simulink model "test_on_intes_cross2018_TestCase"  (R2018b)
settings: Solver=ode1  StartTime=0.0  StopTime=0  FixedStep=0.01  RelTol=1e-3
PostLoadFcn:
  | , if any(exist('dsrtsu_mdlpostloadfcn', 'file') == [2, 3, 6]), try dsrtsu_mdlpostloadfcn('Execute', bdroot); catch fprintf('Error in PostLoadFcn (dsrtsu_mdlpostloadfcn) for model "%s":\n %s\n', bdroot, lasterr); end, end,
values from neighbouring files (symbols this model uses):
  dt = 0.01    [test_on_intes_cross_Autotest.m]    (also in test_on_intes_cross_Autotest_Full.m)
undefined symbols (not defined in the file or in its folder): d0, v0
Description:
  | Standard RTI1401 template.
  | Supported MATLAB version:  R2018b.
settings Model: Tag=RTI1401  DSRTSU_INTERNAL_RTI_VER=540  DSRTSU_INTERNAL_RTI_TYPE=rti1401  RTICANMMDATA=struct('GeneralSetupData',struct('modelroot','C:\Users\linqi\Desktop\matlab\ACC\CarMaker\src_cm4sl','generalsettings',struct('filesettings',struct('destfolder',struct('Name','RTICANMM_FILES','Check',1),'buildfolder',struct('Name','.','Check',1),'AbsDestfolder',struct('Name','C:\Users\linqi\Desktop\matlab\ACC\CarMaker\src_cm4sl\RTICANMM_FILES'),'AbsBuildfolder',struct('Name','C:\Users\linqi\Desktop\matlab\ACC\CarMaker\src_cm4sl'))),'options',struct('addpaths',1,'rmpaths',1,'addtrcexclusion',logical(1),'cannavigator',struct('checkmonitoring',0),'show_usrtrc',0,'use_usrtrc',0),'advanced',struct('options',ones(1,100)),'MPSetup',{{}},'RTI',struct('Type','RTI1401','Ver','7.12','Date','02-May-2019'),'modelname','','block','untitled'))  DSRTSU_INTERNAL_RTIFPGA=130  Creator=linqi  LastModifiedBy=linqi
settings OptimizationCC: BlockReduction=off  OptimizeBlockIOStorage=off  BufferReuse=off  GlobalBufferReuse=off  ExpressionFolding=off  LocalBlockOutputs=off  OptimizeDataStoreBuffers=off  BusAssignmentInplaceUpdate=off
settings DebuggingCC: LibraryContextMissingDiagnostic=none
settings HardwareCC: ProdBitPerPointer=32  ProdBitPerSizeT=32  ProdBitPerPtrDiffT=32  ProdLargestAtomicInteger=Integer  ProdEndianess=BigEndian  ProdWordSize=32  ProdHWDeviceType=Custom Processor->Custom  TargetIntDivRoundTo=Zero  TargetEndianess=BigEndian  TargetHWDeviceType=Custom Processor->Custom
settings SFSimCC: SimUseLocalCustomCode=off  MATLABDynamicMemAlloc=off
settings RTWCC: SystemTargetFile=rti1401.tlc  MakeCommand=make_rti  TemplateMakefile=rti1401.tmf  Description=dSPACE DS1401 Hardware Platform  RTWUseLocalCustomCode=off
settings CodeAppCC: StateflowObjectComments=on
settings STFCustomTargetCC: ParMdlRefBuildCompliant=on  MatFileLogging=on  SystemTargetFile=rti1401.tlc
settings GRTTargetCC: TargetLangStandard=C89/C90 (ANSI)  CompOptLevelCompliant=off  ConcurrentExecutionCompliant=off  CombineOutputUpdateFcns=off  CPPClassGenCompliant=off  UseToolchainInfoCompliant=off
settings ConfigComp: CovMetricSettings=dswe

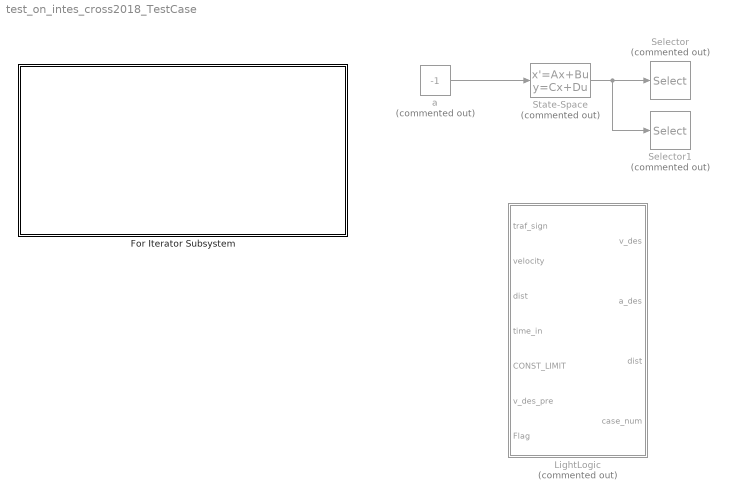
== system test_on_intes_cross2018_TestCase ==
  For Iterator Subsystem : Subsystem  TreatAsAtomicUnit=on
  LightLogic : MATLAB Function  Commented=on  TreatAsAtomicUnit=on
  Selector : Selector  Commented=on  IndexMode=Zero-based  InputPortWidth=2  IndexOptions=Index vector (dialog)  Indices=0  OutputSizes=1
  Selector1 : Selector  Commented=on  IndexMode=Zero-based  InputPortWidth=2  IndexOptions=Index vector (dialog)  Indices=1  OutputSizes=1
  State-Space : StateSpace  Commented=on  A=[0 1;0 0]  B=[0.01/2;1]  C=[1 0;0 1]  D=[0;0]  InitialCondition=[d0;v0]
  a : Constant  Commented=on  Value=-1
  wires:
  a/1 -> State-Space/1
  State-Space/1 -> Selector1/1, Selector/1

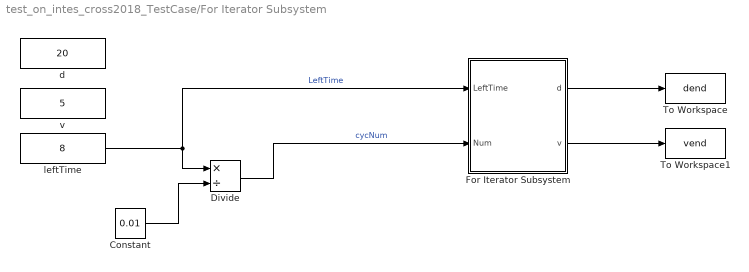
== system test_on_intes_cross2018_TestCase/For Iterator Subsystem ==
  Constant : Constant  Value=0.01  OutDataTypeStr=double
  Divide : Product  Inputs=*/
  For Iterator Subsystem : Subsystem  TreatAsAtomicUnit=on
  To Workspace : ToWorkspace  VariableName=dend  SaveFormat=Timeseries  SampleTime=-1
  To Workspace1 : ToWorkspace  VariableName=vend  SaveFormat=Timeseries  SampleTime=-1
  d : Constant  Value=20  OutDataTypeStr=double
  leftTime : Constant  Value=8  OutDataTypeStr=double
  v : Constant  Value=5  OutDataTypeStr=double
  wires:
  leftTime/1 -> For Iterator Subsystem/1(LeftTime), Divide/1  "LeftTime"
  Constant/1 -> Divide/2
  Divide/1 -> For Iterator Subsystem/2(Num)  "cycNum"
  For Iterator Subsystem/1(d) -> To Workspace/1
  For Iterator Subsystem/2(v) -> To Workspace1/1

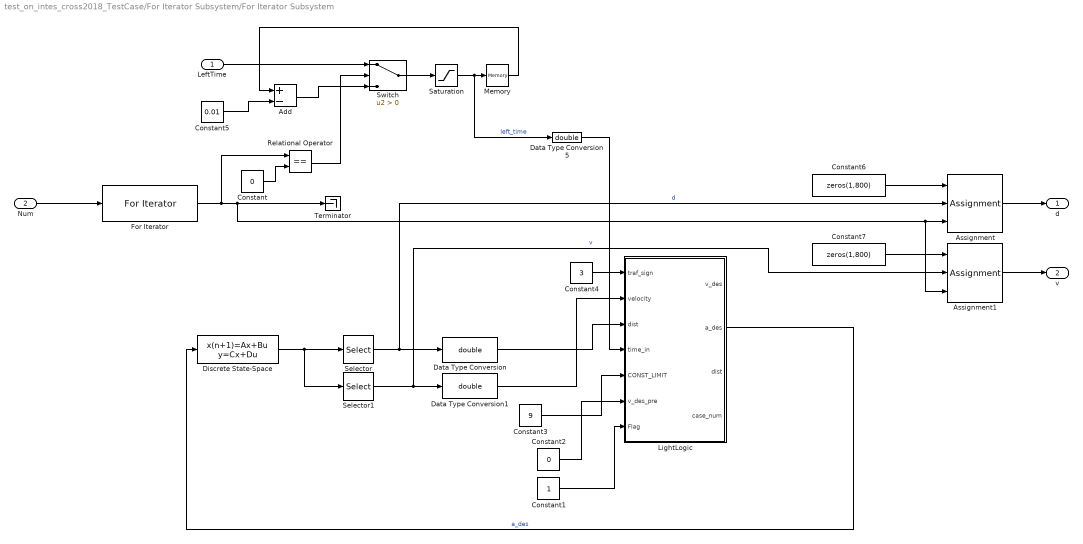
== system test_on_intes_cross2018_TestCase/For Iterator Subsystem/For Iterator Subsystem ==
  LeftTime : Inport
  Num : Inport  Port=2
  Add : Sum  Inputs=+-
  Assignment : Assignment  IndexMode=Zero-based  DiagnosticForDimensions=Warning  IndexOptions=Index vector (port)  Indices=1  OutputSizes=1
  Assignment1 : Assignment  IndexMode=Zero-based  DiagnosticForDimensions=Warning  IndexOptions=Index vector (port)  Indices=1  OutputSizes=1
  Constant : Constant  Value=0
  Constant1 : Constant  OutDataTypeStr=double
  Constant2 : Constant  Value=0  OutDataTypeStr=double
  Constant3 : Constant  Value=9  OutDataTypeStr=double
  Constant4 : Constant  Value=3  OutDataTypeStr=double
  Constant5 : Constant  Value=0.01
  Constant6 : Constant  Value=zeros(1,800)
  Constant7 : Constant  Value=zeros(1,800)
  Data Type Conversion : DataTypeConversion  OutDataTypeStr=double
  Data Type Conversion1 : DataTypeConversion  OutDataTypeStr=double
  Data Type Conversion5 : DataTypeConversion  OutDataTypeStr=double
  Discrete State-Space : DiscreteStateSpace  A=[1 -dt;0 1]  B=[-0.5*dt^2;dt]  C=[1 0;0 1]  D=[0;0]  InitialCondition=[d0;v0]  SampleTime=-1
  For Iterator : ForIterator  IterationSource=external  IndexMode=Zero-based
  LightLogic : MATLAB Function  TreatAsAtomicUnit=on
  Memory : Memory  InheritSampleTime=on
  Relational Operator : RelationalOperator  Operator===  OutDataTypeStr=boolean  RndMeth=Simplest
  Saturation : Saturate  UpperLimit=40  LowerLimit=0
  Selector : Selector  IndexMode=Zero-based  InputPortWidth=2  IndexOptions=Index vector (dialog)  Indices=0  OutputSizes=1
  Selector1 : Selector  IndexMode=Zero-based  InputPortWidth=2  IndexOptions=Index vector (dialog)  Indices=1  OutputSizes=1
  Switch : Switch  Criteria=u2 > Threshold
  Terminator : Terminator
  d : Outport
  v : Outport  Port=2
  wires:
  LightLogic/2(a_des) -> Discrete State-Space/1  "a_des"
  Discrete State-Space/1 -> Selector1/1, Selector/1
  Selector/1 -> Assignment/2, Data Type Conversion/1  "d"
  Constant4/1 -> LightLogic/1(traf_sign)
  Data Type Conversion5/1 -> LightLogic/4(time_in)
  Constant3/1 -> LightLogic/5(CONST_LIMIT)
  Constant1/1 -> LightLogic/7(Flag)
  Constant2/1 -> LightLogic/6(v_des_pre)
  Num/1 -> For Iterator/1
  Constant/1 -> Relational Operator/2
  Relational Operator/1 -> Switch/2
  LeftTime/1 -> Switch/1
  Constant5/1 -> Add/2
  Add/1 -> Switch/3
  Memory/1 -> Add/1
  Switch/1 -> Saturation/1
  Saturation/1 -> Data Type Conversion5/1, Memory/1  "left_time"
  Data Type Conversion/1 -> LightLogic/3("dist ")
  Data Type Conversion1/1 -> LightLogic/2(velocity)
  Constant6/1 -> Assignment/1
  Assignment/1 -> d/1
  Constant7/1 -> Assignment1/1
  For Iterator/1 -> Relational Operator/1, Assignment1/3, Assignment/3, Terminator/1
  Selector1/1 -> Assignment1/2, Data Type Conversion1/1  "v"
  Assignment1/1 -> v/1

== matlab function test_on_intes_cross2018_TestCase/For Iterator Subsystem/For Iterator Subsystem/LightLogic ==
  data: v_des output; a_des output; traf_sign input; velocity input; dist input; time_in input; CONST_LIMIT input; dist output; v_des_pre input; case_num output; Flag input
function [v_des,a_des,dist,case_num] = intesec_cross( traf_sign, velocity, dist, time_in,CONST_LIMIT,v_des_pre,Flag)  
%% this is a function that provide desired velocity, and distance to traffic light;
    % input: trafic_sign with green = 0; red = 1; yellow = 2;
    %        velocity in unit of kph;
    %        dist, and time is distance(m) to cross, and traffic time left
    %        CONST_LIMIT is velocity limit at cross, which is a reference CONSTANT velocity from
    %        ACC module.
    %        v_des_pre preseve previous v_des for next step use.
    
    % output: desired velocity for ACC module, in unit of kph;
    %         dist is distance(m) to front cross;
   
    case_num = 0;
    time = time_in;
    green = 1;
    red = 3;
    yellow = 2;
%     if time == 2
%         a_des = 0;
%          v_des = 0;
%     end
    
    if (Flag == 0)
        v_des = 100;
        a_des = 0;
        dist = 100;
        case_num = 0;
        return;
    end
    
    if dist < 0
        if traf_sign == green
            dist = 200;
        else
            dist = 0;
        end
    end
    
   
    
    
    if (Flag == 1)

        v = velocity;

        if traf_sign == green
            time = time + 3;
        elseif traf_sign == yellow
            traf_sign = green;
        end

        switch traf_sign
            case green
                T_ACC = dist / (v + 0.0001);
                T = time;
                a = 2 * (dist - v * T) / (T^2 + 0.0001);
                v_temp = v + a * T;
                
                if dist == 200
                    v_des = 15;
                    a_des = 0;
                    case_num = 0;
                    return;
                end
                
                if T_ACC < T % green time is long enough
                    if v > CONST_LIMIT %
                        a0 =  (CONST_LIMIT^2 - v^2) / (2*dist + 0.001);
                        a0 = max(a0,-1);
                        vt = sqrt(max(0,v^2 + 2 * a0 * dist));
                        t0 = (vt - v) / (a0);
                        
                        if t0 <= T % decelerate to vt is OK
                            v_des = vt % (v + t0 * a0);
                            a_des = a0;
                            case_num = 1;
                        else 
                            v_des = v + T * a0;
                            a_des = a0;
                            case_num = 2;
                        end
                    else % green 
                        v_des = CONST_LIMIT;
                        a_des = (CONST_LIMIT - v)/T;
                        case_num = 3;
                    end
                    
                else % ( T_ACC >= T)
                    if ((a >= 0) && (a < 1) && (v_temp <= CONST_LIMIT))
                        v_des = CONST_LIMIT;
                        a_des = a;
                        case_num = 4;
                    else
                        v_des  = 0;
                        a_des = -v^2 / (2 * dist);
                        case_num = 5;
                    end
                end

            case red
                
                    if (dist < 4) && (v < 1)
                        a_des = 0.25 * dist - 1;
                        v_des = 0;
                        case_num = 12;
                        
                    else
                        T = time;
                        T_ACC = dist / (v + 0.0001);
                        a = 2 * (dist - v * T) / (T+0.001)^2;
                        v_temp = v + a * T;

                        if T_ACC < T
                            a0 = -v^2 / (2 * dist);
                            t0 = -v / a0;
                            if t0 < time
                                v_des = 0;
                                a_des = -v^2 / (2 * dist+ 0.01);
                                case_num = 7;
                            else
                                v_des = v_temp;
                                a_des = a;
                                case_num = 8;
                            end 
  
                        else % (T_ACC > T)
                            if (v_temp < CONST_LIMIT)
                                v_des = v_temp;
                                a_des = a;
                                case_num = 9;
                            else
                                v_des = CONST_LIMIT;
                                a_des = (CONST_LIMIT - v) / T;
                                case_num = 10;
                            end
                             
                        end
                    end
                    
               

            otherwise
                v_des = CONST_LIMIT;
                a_des = 0;
                case_num = 11;
        end
        
    else
        v_des = 100;
        a_des = 100;
        dist = 100;
        case_num = 0;
         
    end
end

== matlab function test_on_intes_cross2018_TestCase/LightLogic ==
  data: v_des output; a_des output; traf_sign input; velocity input; dist input; time_in input; CONST_LIMIT input; dist output; v_des_pre input; case_num output; Flag input
function [v_des,a_des,dist,case_num] = intesec_cross( traf_sign, velocity, dist, time_in,CONST_LIMIT,v_des_pre,Flag)  
%% this is a function that provide desired velocity, and distance to traffic light;
    % input: trafic_sign with green = 0; red = 1; yellow = 2;
    %        velocity in unit of kph;
    %        dist, and time is distance(m) to cross, and traffic time left
    %        CONST_LIMIT is velocity limit at cross, which is a reference CONSTANT velocity from
    %        ACC module.
    %        v_des_pre preseve previous v_des for next step use.
    
    % output: desired velocity for ACC module, in unit of kph;
    %         dist is distance(m) to front cross;
   
    case_num = 0;
    time = time_in;
    green = 1;
    red = 3;
    yellow = 2;
%     if time == 2
%         a_des = 0;
%          v_des = 0;
%     end
    
    if (Flag == 0)
        v_des = 100;
        a_des = 0;
        dist = 100;
        case_num = 0;
        return;
    end
    
    if dist < 0
        if traf_sign == green
            dist = 200;
        else
            dist = 0;
        end
    end
    
   
    
    
    if (Flag == 1)

        v = velocity;

        if traf_sign == green
            time = time + 3;
        elseif traf_sign == yellow
            traf_sign = green;
        end

        switch traf_sign
            case green
                T_ACC = dist / (v + 0.0001);
                T = time;
                a = 2 * (dist - v * T) / (T^2 + 0.0001);
                v_temp = v + a * T;
                
                if dist == 200
                    v_des = 15;
                    a_des = 0;
                    case_num = 0;
                    return;
                end
                
                if T_ACC < T % green time is long enough
                    if v > CONST_LIMIT %
                        a0 =  (CONST_LIMIT^2 - v^2) / (2*dist + 0.001);
                        a0 = max(a0,-1);
                        vt = sqrt(max(0,v^2 + 2 * a0 * dist));
                        t0 = (vt - v) / (a0);
                        
                        if t0 <= T % decelerate to vt is OK
                            v_des = vt % (v + t0 * a0);
                            a_des = a0;
                            case_num = 1;
                        else 
                            v_des = v + T * a0;
                            a_des = a0;
                            case_num = 2;
                        end
                    else % green 
                        v_des = CONST_LIMIT;
                        a_des = (CONST_LIMIT - v)/T;
                        case_num = 3;
                    end
                    
                else % ( T_ACC >= T)
                    if ((a >= 0) && (a < 1) && (v_temp <= CONST_LIMIT))
                        v_des = CONST_LIMIT;
                        a_des = a;
                        case_num = 4;
                    else
                        v_des  = 0;
                        a_des = -v^2 / (2 * dist);
                        case_num = 5;
                    end
                end

            case red
                
                    if (dist < 4) && (v < 1)
                        a_des = 0.25 * dist - 1;
                        v_des = 0;
                        case_num = 12;
                        
                    else
                        T = time;
                        T_ACC = dist / (v + 0.0001);
                        a = 2 * (dist - v * T) / (T+0.001)^2;
                        v_temp = v + a * T;

                        if T_ACC < T
                            a0 = -v^2 / (2 * dist);
                            t0 = -v / a0;
                            if t0 < time
                                v_des = 0;
                                a_des = -v^2 / (2 * dist+ 0.01);
                                case_num = 7;
                            else
                                v_des = v_temp;
                                a_des = a;
                                case_num = 8;
                            end 
  
                        else % (T_ACC > T)
                            if (v_temp < CONST_LIMIT)
                                v_des = v_temp;
                                a_des = a;
                                case_num = 9;
                            else
                                v_des = CONST_LIMIT;
                                a_des = (CONST_LIMIT - v) / T;
                                case_num = 10;
                            end
                             
                        end
                    end
                    
               

            otherwise
                v_des = CONST_LIMIT;
                a_des = 0;
                case_num = 11;
        end
        
    else
        v_des = 100;
        a_des = 100;
        dist = 100;
        case_num = 0;
         
    end
end
